simulink model "main_sim_adapt"  (Simulink 7.2)
settings: Solver=ode2  SolverMode=SingleTasking  StartTime=0.0  StopTime=tsim_max  FixedStep=dtsim  RelTol=1e-3
StopFcn:
  | %mkplt
undefined symbols (not defined in the file): aero_surf_qbar_off, aero_surf_qbar_on, assertion_time, att_type, att_type_numbers, bb_ellipsoid, bb_params, compute_all_rate_cols, compute_all_vel_cols, constants, cosA, DiscIntNeverNeededParam, dtsim, E_rwy, eow_boundary, full_surf_llim, full_surf_ulim, gain_set, gain_var_struct, in_exsig_vecin, in_exsig_vecout, MACH, MACH_att_fb, MACH_gain_mat, MACH_mass_IC, MACH_pos_IC, MACH_pqr_Bmat_IC, MACH_pqr_IC, MACH_pqr_u_IC, MACH_quat_IC, MACH_throttle_IC, MACH_U_nom_IC, MACH_vel_Bmat_IC, MACH_vel_cvdnom_IC, MACH_vel_IC, MACH_vel_uold_IC, max_LOS_rate, modes, N_rwy, pos, rcs_cvddes_thresh, reset_camcmd_on_entry, sinA, target_pos_IC, target_range_blind, target_range_detect, target_range_homing, target_vel_IC, trac_params, u_llim, u_ulim, use_auto_att_type, use_eow_as_iv, use_nav, use_pos_fltpath_lim, use_throt_estimate, use_variable_mass, use_wind_est, vel, vel_cmd_ramp_time ... (+1)
libraries: simulink x32, mach_lib x26, utility_lib x24, model_lib x15, simulink_need_slupdate x8, models x6
(part 1 of 5)
CloseFcn:
  | rtwprivate ssgencode ModelCloseRequest main
settings Model: Creator=E183308  LastModifiedBy=E183308  ModifiedComment=E700252 -- Tue Nov 11 13:33:23 2003 -- Version 1.2477  TunableVars=MACH_U_nom_IC,MACH_gain_mat,MACH_mass_IC,MACH_pos_IC,MACH_pqr_Bmat_IC,MACH_pqr_u_IC,MACH_quat_IC,MACH_throttle_IC,MACH_vel_Bmat_IC,MACH_vel_IC,MACH_vel_cvdnom_IC,MACH_vel_uold_IC  TunableVarsStorageClass=Auto,Auto,Auto,Auto,Auto,Auto,Auto,Auto,Auto,Auto,Auto,Auto  TunableVarsTypeQualifier=,,,,,,,,,,,  BufferReuse=off
settings DataIOCC: LimitDataPoints=off  SaveOutput=off  SaveTime=off  SignalLoggingName=sigsOut
settings OptimizationCC: BlockReduction=off  BooleanDataType=off  BufferReuse=off  EnforceIntegerDowncast=off  FoldNonRolledExpr=off  InitFltsAndDblsToZero=on
settings DebuggingCC: SaveWithParameterizedLinksMsg=none  SignalResolutionControl=TryResolveAllWithWarning  SolverPrmCheckMsg=none  InheritedTsInSrcMsg=none  MultiTaskDSMMsg=warning  MultiTaskCondExecSysMsg=none  StrictBusMsg=ErrorLevel1
settings HardwareCC: TargetEndianess=LittleEndian  TargetHWDeviceType=MATLAB Host  ProdEqTarget=off
settings SFSimCC: SFSimEcho=off
settings RTWCC: SystemTargetFile=rtwsfcn.tlc  TemplateMakefile=rtwsfcn_default_tmf  Description=S-function Target  ProcessScript=rtwsfcn_make_rtw_hook  IncludeERTFirstTime=on
settings STFCustomTargetCC: TargetFcnLib=ansi_tfl_tmw.mat  ModelReferenceCompliant=off  SystemTargetFile=rtwsfcn.tlc
settings CustomProperty: Value=on

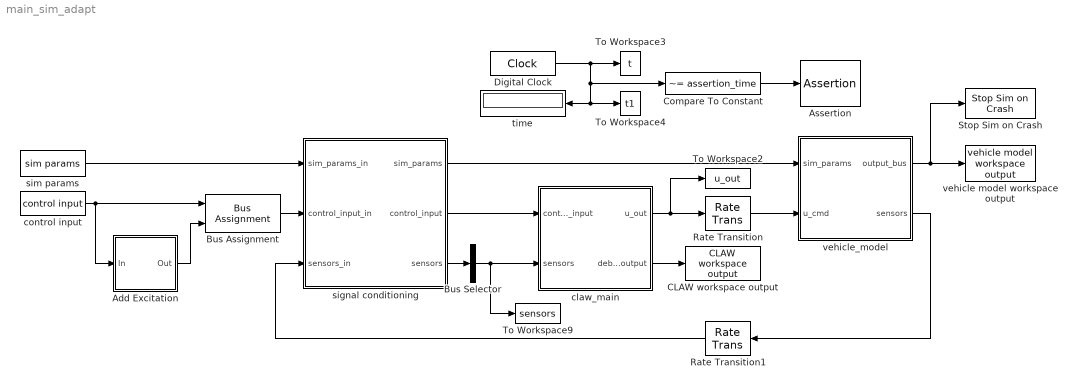
== system main_sim_adapt ==
  Add Excitation : Subsystem
  Assertion : Assertion  Enabled=on  AssertionFailFcn=assertioncb  StopWhenAssertionFail=off
  Bus Assignment : BusAssignment  AssignedSignals=command
  Bus Selector : BusSelector  OutputSignals=pqr,NED_dot,latlonh,e,accels_cg,nav_ok,u_meas,NED_wind,seeker  OutputAsBus=on
  CLAW workspace output : mach_lib/CLAW workspace output  SystemSampleTime=-1
  Compare To Constant : simulink/Logic and Bit Operations/Compare To Constant  SystemSampleTime=-1  relop=~=  const=assertion_time  LogicOutDataTypeMode=boolean  ZeroCross=off
  Digital Clock : DigitalClock  SampleTime=dtsim
  Rate Transition : RateTransition  X0=MACH_U_nom_IC
  Rate Transition1 : RateTransition  Orientation=left  OutPortSampleTime=MACH.dt
  Stop Sim on Crash : mach_lib/Stop Sim on Crash  SystemSampleTime=-1
  To Workspace2 : ToWorkspace  VariableName=u_out  SampleTime=MACH.dt  SaveFormat=Array
  To Workspace3 : ToWorkspace  VariableName=t  SampleTime=dtsim  SaveFormat=Array
  To Workspace4 : ToWorkspace  VariableName=t1  SampleTime=MACH.dt  SaveFormat=Array
  To Workspace9 : ToWorkspace  VariableName=sensors  SampleTime=MACH.dt  SaveFormat=Array
      settings: MaxDataPoints=1
  claw_main : Subsystem  AncestorBlock=mach_lib/claw_main  TreatAsAtomicUnit=on  SystemSampleTime=MACH.dt
  control input : mach_lib/control input  SystemSampleTime=MACH.dt
  signal conditioning : Subsystem
  sim params : mach_lib/sim params  SystemSampleTime=-1
  time : Display
  vehicle model workspace output : mach_lib/vehicle model workspace output  SystemSampleTime=-1
  vehicle_model : Subsystem  TreatAsAtomicUnit=on
  wires:
  Digital Clock/1 -> To Workspace3/1, time/1, To Workspace4/1, Compare To Constant/1
  claw_main/1(u_out) -> Rate Transition/1, To Workspace2/1
  vehicle_model/2(sensors) -> Rate Transition1/1
  claw_main/2(debug_output) -> CLAW workspace output/1
  Rate Transition/1 -> vehicle_model/2(u_cmd)
  Bus Selector/1 -> To Workspace9/1, claw_main/2(sensors)
  vehicle_model/1(output_bus) -> vehicle model workspace output/1, Stop Sim on Crash/1
  Rate Transition1/1 -> signal conditioning/3(sensors_in)
  signal conditioning/3(sensors) -> Bus Selector/1
  signal conditioning/2(control_input) -> claw_main/1(control_input)
  control input/1 -> Bus Assignment/1, Add Excitation/1(In)
  sim params/1 -> signal conditioning/1(sim_params_in)
  signal conditioning/1(sim_params) -> vehicle_model/1(sim_params)
  Compare To Constant/1 -> Assertion/1
  Bus Assignment/1 -> signal conditioning/2(control_input_in)
  Add Excitation/1(Out) -> Bus Assignment/2

== system main_sim_adapt/Add Excitation ==
  In : Inport
  Bus Selector1 : BusSelector  OutputSignals=command
      settings: CopyFcn=set_param(gcbh,'ShowName','off','CopyFcn','')
  Demux : Demux  Outputs=[1 1 1 1]
      settings: CopyFcn=set_param(gcbh,'ShowName','off','CopyFcn','')
  Excitation  Signal : Subsystem
  Mux : Mux
      settings: CopyFcn=set_param(gcbh,'ShowName','off','CopyFcn','')
  Rate Transition2 : RateTransition  OutPortSampleTime=MACH.dt
  Step : Step  SampleTime=MACH.dt
  Sum : Sum  Inputs=|++  OutDataType=sfix(16)  OutScaling=2^0
      settings: CopyFcn=set_param(gcbh,'ShowName','off','CopyFcn','')
  Out : Outport
  wires:
  Bus Selector1/1 -> Demux/1  "<command>"
  Demux/1 -> Mux/1
  Demux/3 -> Mux/3
  Demux/2 -> Sum/1
  Sum/1 -> Mux/2
  Step/1 -> Excitation  Signal/Enable
  Excitation  Signal/1(exsig) -> Rate Transition2/1
  Rate Transition2/1 -> Sum/2
  Demux/4 -> Mux/4
  In/1 -> Bus Selector1/1
  Mux/1 -> Out/1

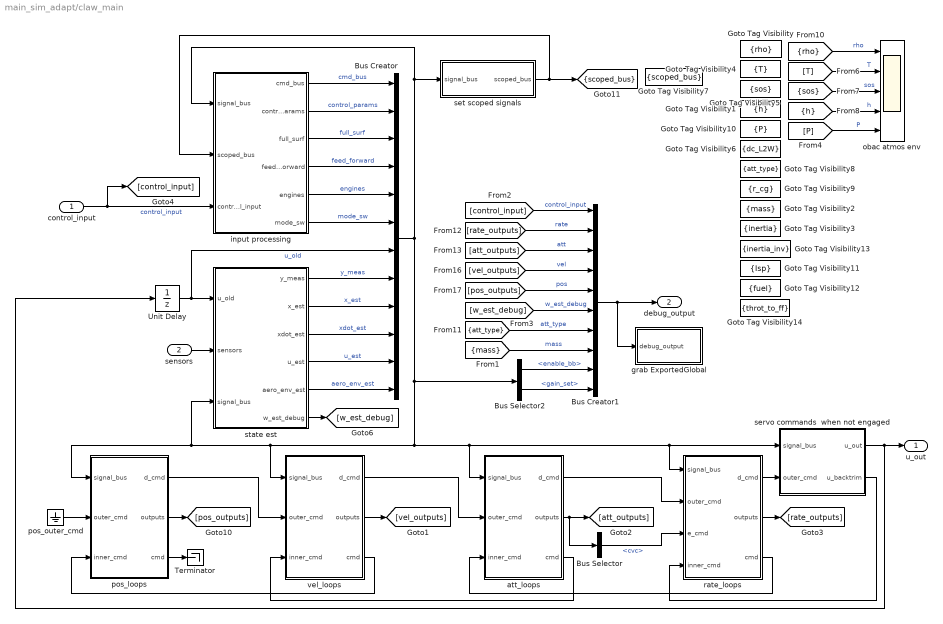
== system main_sim_adapt/claw_main ==
  control_input : Inport  OutDataType=sfix(16)  OutScaling=2^0
      settings: BusObject=control_input_bus
  sensors : Inport  Port=2  OutDataType=sfix(16)  OutScaling=2^0
  Bus Creator : BusCreator  Inputs=12
  Bus Creator1 : BusCreator  Inputs=10
      settings: BusObject=CLAW_DEBUG_OUTPUT_BUS
  Bus Selector : BusSelector  OutputSignals=cvc
  Bus Selector2 : BusSelector  OutputSignals=control_params.enable_bb,control_params.gain_set
  Goto Tag Visibility : GotoTagVisibility  GotoTag=rho
  Goto Tag Visibility1 : GotoTagVisibility  GotoTag=h
  Goto Tag Visibility10 : GotoTagVisibility  GotoTag=P
  Goto Tag Visibility11 : GotoTagVisibility  GotoTag=Isp
  Goto Tag Visibility12 : GotoTagVisibility  GotoTag=fuel
  Goto Tag Visibility13 : GotoTagVisibility  GotoTag=inertia_inv
  Goto Tag Visibility14 : GotoTagVisibility  GotoTag=throt_to_ff
  Goto Tag Visibility2 : GotoTagVisibility  GotoTag=mass
  Goto Tag Visibility3 : GotoTagVisibility  GotoTag=inertia
  Goto Tag Visibility4 : GotoTagVisibility  GotoTag=T
  Goto Tag Visibility5 : GotoTagVisibility  GotoTag=sos
  Goto Tag Visibility6 : GotoTagVisibility  GotoTag=dc_L2W
  Goto Tag Visibility7 : GotoTagVisibility  GotoTag=scoped_bus
  Goto Tag Visibility8 : GotoTagVisibility  GotoTag=att_type
  Goto Tag Visibility9 : GotoTagVisibility  GotoTag=r_cg
  Terminator : Terminator
  Unit Delay : UnitDelay  X0=MACH_U_nom_IC  SampleTime=-1
  att_loops : Subsystem
  grab ExportedGlobal : Subsystem
  input processing : Subsystem
  obac atmos env : Scope  NumInputPorts=5
      settings: YMin=-5~-5~-5~-5~-5  YMax=5~5~5~5~5  SaveName=ScopeData2
  pos_loops : Subsystem
      settings: RTWSystemCode=Function
  pos_outer_cmd : Ground
  rate_loops : Subsystem
      settings: RTWSystemCode=Function
  servo commands  when not engaged : Subsystem
  set scoped signals : Subsystem
  state est : Subsystem
  vel_loops : Subsystem
      settings: RTWSystemCode=Function
  u_out : Outport  OutDataType=sfix(16)  OutScaling=2^0
  debug_output : Outport  Port=2  OutDataType=sfix(16)  OutScaling=2^0
  tag scope: scoped_bus=scoped
  wires:
  input processing/6(mode_sw) -> Bus Creator/6  "mode_sw"
  input processing/5(engines) -> Bus Creator/5  "engines"
  pos_loops/2(outputs) -> [pos_outputs]
  [pos_outputs] -> Bus Creator1/5  "pos"
  [vel_outputs] -> Bus Creator1/4  "vel"
  [att_outputs] -> Bus Creator1/3  "att"
  [rate_outputs] -> Bus Creator1/2  "rate"
  att_loops/1(d_cmd) -> rate_loops/2(outer_cmd)
  vel_loops/1(d_cmd) -> att_loops/2(outer_cmd)
  rate_loops/1(d_cmd) -> servo commands  when not engaged/2(outer_cmd)
  Bus Creator/1 -> att_loops/1(signal_bus), rate_loops/1(signal_bus), servo commands  when not engaged/1(signal_bus), vel_loops/1(signal_bus), pos_loops/1(signal_bus), state est/3(signal_bus), Bus Selector2/1, input processing/1(signal_bus), set scoped signals/1(signal_bus)
  pos_loops/3(cmd) -> Terminator/1
  att_loops/3(cmd) -> vel_loops/3(inner_cmd)
  rate_loops/3(cmd) -> att_loops/3(inner_cmd)
  pos_loops/1(d_cmd) -> vel_loops/2(outer_cmd)
  vel_loops/2(outputs) -> [vel_outputs]
  att_loops/2(outputs) -> [att_outputs], Bus Selector/1
  rate_loops/2(outputs) -> [rate_outputs]
  Bus Creator1/1 -> debug_output/1, grab ExportedGlobal/1(debug_output)
  Unit Delay/1 -> state est/1(u_old), Bus Creator/7  "u_old"
  sensors/1 -> state est/2(sensors)
  vel_loops/3(cmd) -> pos_loops/3(inner_cmd)
  servo commands  when not engaged/2(u_backtrim) -> rate_loops/4(inner_cmd)
  state est/4(u_est) -> Bus Creator/11  "u_est"
  state est/3(xdot_est) -> Bus Creator/10  "xdot_est"
  state est/2(x_est) -> Bus Creator/9  "x_est"
  state est/1(y_meas) -> Bus Creator/8  "y_meas"
  servo commands  when not engaged/1(u_out) -> u_out/1, Unit Delay/1
  pos_outer_cmd/1 -> pos_loops/2(outer_cmd)
  state est/6(w_est_debug) -> [w_est_debug]
  [w_est_debug] -> Bus Creator1/6  "w_est_debug"
  [att_type] -> Bus Creator1/7  "att_type"
  input processing/2(control_params) -> Bus Creator/2  "control_params"
  [h] -> obac atmos env/4  "h"
  [sos] -> obac atmos env/3  "sos"
  [T] -> obac atmos env/2  "T"
  [rho] -> obac atmos env/1  "rho"
  [P] -> obac atmos env/5  "P"
  state est/5(aero_env_est) -> Bus Creator/12  "aero_env_est"
  input processing/3(full_surf) -> Bus Creator/3  "full_surf"
  input processing/4(feed_forward) -> Bus Creator/4  "feed_forward"
  set scoped signals/1(scoped_bus) -> [scoped_bus], input processing/2(scoped_bus)
  [mass] -> Bus Creator1/8  "mass"
  Bus Selector2/1 -> Bus Creator1/9  "<enable_bb>"
  Bus Selector2/2 -> Bus Creator1/10  "<gain_set>"
  control_input/1 -> input processing/3(control_input), [control_input]  "control_input"
  input processing/1(cmd_bus) -> Bus Creator/1  "cmd_bus"
  [control_input] -> Bus Creator1/1  "control_input"
  Bus Selector/1 -> rate_loops/3(e_cmd)  "<cvc>"

== system main_sim_adapt/signal conditioning ==
  sim_params_in : Inport  OutDataType=sfix(16)  OutScaling=2^0
  control_input_in : Inport  Port=2  OutDataType=sfix(16)  OutScaling=2^0
  sensors_in : Inport  Port=3  OutDataType=sfix(16)  OutScaling=2^0
  Bus Assignment : BusAssignment  AssignedSignals=full_surf.full_surf_pref
  Bus Selector : BusSelector  OutputSignals=full_surf.full_surf_pref
  Compare To Constant : simulink/Logic and Bit Operations/Compare To Constant  SystemSampleTime=-1  relop=>=  const=0  LogicOutDataTypeMode=boolean  ZeroCross=off
  Compare To Constant1 : simulink/Logic and Bit Operations/Compare To Constant  SystemSampleTime=-1  relop=<=  const=5  LogicOutDataTypeMode=boolean  ZeroCross=off
  Constant : Constant  Value=360  OutDataType=sfix(16)  OutScaling=2^0
  Digital Clock : DigitalClock  SampleTime=MACH.dt
  Gain : Gain  Gain=0  ParameterDataType=sfix(16)  ParameterScaling=2^0  OutDataType=sfix(16)  OutScaling=2^0
  Logical Operator : Logic  AllPortsSameDT=off
  Product : Product  OutDataType=sfix(16)  OutScaling=2^0  RndMeth=Zero
  Sine Wave : Sin  TimeSource=Use external signal  Amplitude=5  Frequency=2*pi  SampleTime=0
  Sum : Sum  Inputs=|++  OutDataType=sfix(16)  OutScaling=2^0
  Sum1 : Sum  Inputs=|+-  OutDataType=sfix(16)  OutScaling=2^0
  get RIE : Selector  InputPortWidth=MACH.num_u  IndexOptions=Index vector (dialog)  Indices=MACH.vane_idx(1)  OutputSizes=1
  set RIE : Assignment  IndexOptions=Index vector (dialog)  Indices=MACH.vane_idx(1)  OutputSizes=[1 1]
  sim_params : Outport  OutDataType=sfix(16)  OutScaling=2^0
  control_input : Outport  Port=2  OutDataType=sfix(16)  OutScaling=2^0
  sensors : Outport  Port=3  OutDataType=sfix(16)  OutScaling=2^0
  wires:
  sim_params_in/1 -> sim_params/1
  control_input_in/1 -> Bus Assignment/1, Bus Selector/1
  sensors_in/1 -> sensors/1
  set RIE/1 -> Bus Assignment/2
  Sum/1 -> set RIE/2
  Bus Selector/1 -> set RIE/1, get RIE/1  "<full_surf_pref>"
  get RIE/1 -> Sum/1
  Digital Clock/1 -> Sum1/1
  Constant/1 -> Sum1/2
  Sum1/1 -> Sine Wave/1, Compare To Constant/1, Compare To Constant1/1
  Compare To Constant/1 -> Logical Operator/1
  Compare To Constant1/1 -> Logical Operator/2
  Logical Operator/1 -> Product/2
  Sine Wave/1 -> Product/1
  Product/1 -> Gain/1
  Bus Assignment/1 -> control_input/1
  Gain/1 -> Sum/2

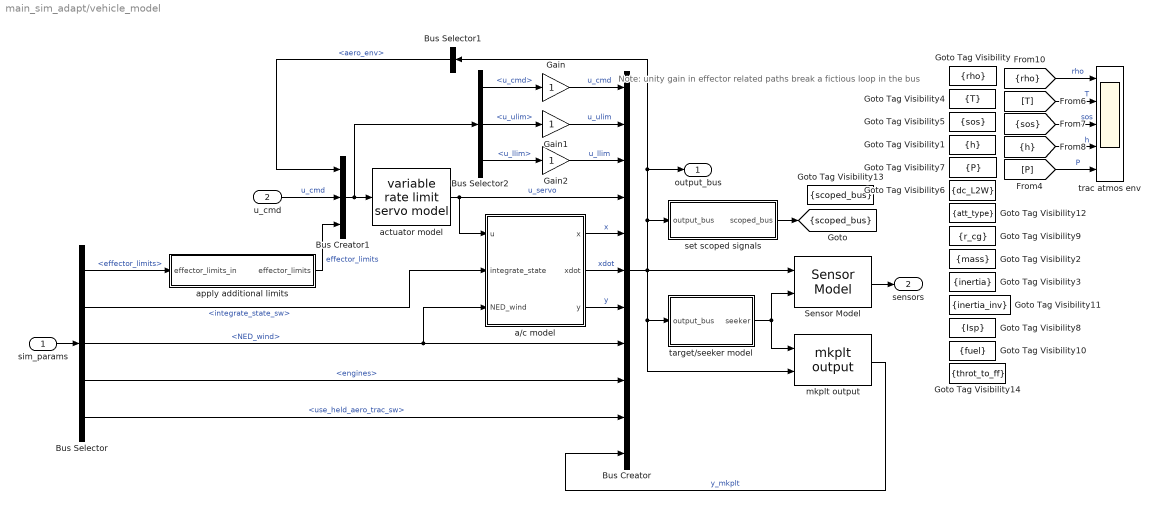
== system main_sim_adapt/vehicle_model ==
  note: Note: unity gain in effector related paths
      | break a fictious loop in the bus
  sim_params : Inport  OutDataType=sfix(16)  OutScaling=2^0
  u_cmd : Inport  Port=2  OutDataType=sfix(16)  OutScaling=2^0
  Bus Creator : BusCreator  Inputs=11
  Bus Creator1 : BusCreator  Inputs=3
  Bus Selector : BusSelector  OutputSignals=effector_limits,integrate_state_sw,NED_wind,engines,use_held_aero_trac_sw
  Bus Selector1 : BusSelector  Orientation=left  OutputSignals=y.aero_env
  Bus Selector2 : BusSelector  OutputSignals=u_cmd,effector_limits.u_ulim,effector_limits.u_llim
  Gain : Gain  ParameterDataType=sfix(16)  ParameterScaling=2^0  OutDataType=sfix(16)  OutScaling=2^0
  Gain1 : Gain  ParameterDataType=sfix(16)  ParameterScaling=2^0  OutDataType=sfix(16)  OutScaling=2^0
  Gain2 : Gain  ParameterDataType=sfix(16)  ParameterScaling=2^0  OutDataType=sfix(16)  OutScaling=2^0
  Goto Tag Visibility : GotoTagVisibility  GotoTag=rho
  Goto Tag Visibility1 : GotoTagVisibility  GotoTag=h
  Goto Tag Visibility10 : GotoTagVisibility  GotoTag=fuel
  Goto Tag Visibility11 : GotoTagVisibility  GotoTag=inertia_inv
  Goto Tag Visibility12 : GotoTagVisibility  GotoTag=att_type
  Goto Tag Visibility13 : GotoTagVisibility  GotoTag=scoped_bus
  Goto Tag Visibility14 : GotoTagVisibility  GotoTag=throt_to_ff
  Goto Tag Visibility2 : GotoTagVisibility  GotoTag=mass
  Goto Tag Visibility3 : GotoTagVisibility  GotoTag=inertia
  Goto Tag Visibility4 : GotoTagVisibility  GotoTag=T
  Goto Tag Visibility5 : GotoTagVisibility  GotoTag=sos
  Goto Tag Visibility6 : GotoTagVisibility  GotoTag=dc_L2W
  Goto Tag Visibility7 : GotoTagVisibility  GotoTag=P
  Goto Tag Visibility8 : GotoTagVisibility  GotoTag=Isp
  Goto Tag Visibility9 : GotoTagVisibility  GotoTag=r_cg
  Sensor Model : model_lib/Sensor Model  SystemSampleTime=-1
  a/c model : Subsystem
  actuator model : model_lib/variable rate limit servo model  SystemSampleTime=-1
  apply additional limits : Subsystem
  mkplt output : model_lib/mkplt output  SystemSampleTime=-1
  set scoped signals : Subsystem
  target/seeker model : Subsystem
  trac atmos env : Scope  NumInputPorts=5
      settings: YMin=-5~-5~-5~-5~-5  YMax=5~5~5~5~5
  output_bus : Outport  OutDataType=sfix(16)  OutScaling=2^0
  sensors : Outport  Port=2  OutDataType=sfix(16)  OutScaling=2^0
  tag scope: scoped_bus=scoped
  wires:
  actuator model/1 -> a/c model/1(u), Bus Creator/4  "u_servo"
  Sensor Model/1 -> sensors/1
  Bus Selector/3 -> Bus Creator/8, a/c model/3(NED_wind)  "<NED_wind>"
  [h] -> trac atmos env/4  "h"
  [sos] -> trac atmos env/3  "sos"
  [T] -> trac atmos env/2  "T"
  [rho] -> trac atmos env/1  "rho"
  [P] -> trac atmos env/5  "P"
  target/seeker model/1(seeker) -> Sensor Model/2, mkplt output/1
  a/c model/1(x) -> Bus Creator/5  "x"
  a/c model/2(xdot) -> Bus Creator/6  "xdot"
  a/c model/3(y) -> Bus Creator/7  "y"
  Bus Creator/1 -> set scoped signals/1(output_bus), output_bus/1, Bus Selector1/1, target/seeker model/1(output_bus), mkplt output/2, Sensor Model/1
  sim_params/1 -> Bus Selector/1
  set scoped signals/1(scoped_bus) -> [scoped_bus]
  Bus Selector/4 -> Bus Creator/9  "<engines>"
  mkplt output/1 -> Bus Creator/11  "y_mkplt"
  Bus Selector/5 -> Bus Creator/10  "<use_held_aero_trac_sw>"
  Bus Creator1/1 -> actuator model/1, Bus Selector2/1
  Bus Selector1/1 -> Bus Creator1/1  "<aero_env>"
  u_cmd/1 -> Bus Creator1/2  "u_cmd"
  Bus Selector2/1 -> Gain/1  "<u_cmd>"
  Bus Selector2/2 -> Gain1/1  "<u_ulim>"
  Bus Selector2/3 -> Gain2/1  "<u_llim>"
  Gain/1 -> Bus Creator/1  "u_cmd"
  Gain1/1 -> Bus Creator/2  "u_ulim"
  Gain2/1 -> Bus Creator/3  "u_llim"
  Bus Selector/2 -> a/c model/2(integrate_state)  "<integrate_state_sw>"
  Bus Selector/1 -> apply additional limits/1(effector_limits_in)  "<effector_limits>"
  apply additional limits/1(effector_limits) -> Bus Creator1/3  "effector_limits"

== system main_sim_adapt/Add Excitation/Excitation  Signal ==
  Enable : EnablePort  StatesWhenEnabling=reset  ShowOutputPort=on
  Integrator : Integrator  ExternalReset=falling
  Lookup Table1 : Lookup  InputValues=in_exsig_vecin  Table=in_exsig_vecout  LookUpMeth=Use Input Above  OutDataType=sfix(16)  OutScaling=2^0
  excitaiton output sig : Scope
      settings: TimeRange=45  YMin=-0.05  YMax=0.05  SaveName=ScopeData5
  excitation input sig : Scope
      settings: TimeRange=45  YMin=15  YMax=22  SaveName=ScopeData10
  exsig : Outport  OutDataType=sfix(16)  OutScaling=2^0  OutputWhenDisabled=reset  InitialOutput=0
  wires:
  Lookup Table1/1 -> exsig/1, excitaiton output sig/1
  Enable/1 -> Integrator/1, Integrator/2
  Integrator/1 -> Lookup Table1/1, excitation input sig/1

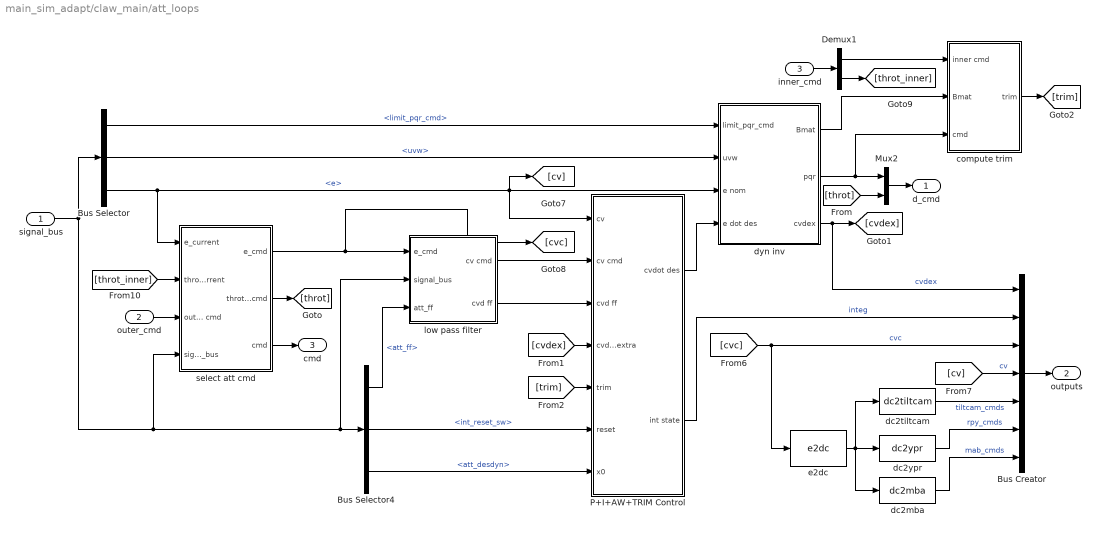
== system main_sim_adapt/claw_main/att_loops ==
  signal_bus : Inport  OutDataType=sfix(16)  OutScaling=2^0
  outer_cmd : Inport  Port=2  OutDataType=sfix(16)  OutScaling=2^0
  inner_cmd : Inport  Port=3  OutDataType=sfix(16)  OutScaling=2^0
  Bus Creator : BusCreator  Inputs=7
  Bus Selector : BusSelector  OutputSignals=control_params.limit_pqr_cmd,x_est.uvw,x_est.e
  Bus Selector4 : BusSelector  OutputSignals=feed_forward.att_ff,mode_sw.int_reset_sw,control_params.att_desdyn
  Demux1 : Demux  Outputs=[ MACH.att_num_u MACH.num_u_throt ]
  Mux2 : Mux  Inputs=2
  P+I+AW+TRIM Control : Subsystem
  compute trim : Subsystem
  dc2mba : utility_lib/dc2mba  SystemSampleTime=-1
  dc2tiltcam : utility_lib/dc2tiltcam  SystemSampleTime=-1
  dc2ypr : utility_lib/dc2ypr  SystemSampleTime=-1
  dyn inv : Subsystem
  e2dc : utility_lib/e2dc  SystemSampleTime=-1
  low pass filter : Subsystem
  select att cmd : Subsystem
  d_cmd : Outport  OutDataType=sfix(16)  OutScaling=2^0
  outputs : Outport  Port=2  OutDataType=sfix(16)  OutScaling=2^0
  cmd : Outport  Port=3  OutDataType=sfix(16)  OutScaling=2^0
  wires:
  Mux2/1 -> d_cmd/1
  [throt] -> Mux2/2
  P+I+AW+TRIM Control/2(int state) -> Bus Creator/2  "integ"
  dyn inv/3(cvdex) -> [cvdex], Bus Creator/1  "cvdex"
  Bus Selector/3 -> select att cmd/1(e_current), dyn inv/3(e nom), [cv], P+I+AW+TRIM Control/1(cv)  "<e>"
  outer_cmd/1 -> select att cmd/3(outer cmd)
  P+I+AW+TRIM Control/1(cvdot des) -> dyn inv/4(e dot des)
  [cvdex] -> P+I+AW+TRIM Control/4(cvdot extra)
  dyn inv/1(Bmat) -> compute trim/2(Bmat)
  [trim] -> P+I+AW+TRIM Control/5(trim)
  signal_bus/1 -> Bus Selector/1, select att cmd/4(signal_bus), Bus Selector4/1, low pass filter/2(signal_bus)
  compute trim/1(trim) -> [trim]
  select att cmd/2(throt_cmd) -> [throt]
  [cvc] -> Bus Creator/3, e2dc/1  "cvc"
  Bus Creator/1 -> outputs/1
  inner_cmd/1 -> Demux1/1
  Demux1/1 -> compute trim/1(inner cmd)
  Demux1/2 -> [throt_inner]
  dc2tiltcam/1 -> Bus Creator/5  "tiltcam_cmds"
  [cv] -> Bus Creator/4  "cv"
  e2dc/1 -> dc2tiltcam/1, dc2ypr/1, dc2mba/1
  dc2ypr/1 -> Bus Creator/6  "rpy_cmds"
  dc2mba/1 -> Bus Creator/7  "mab_cmds"
  Bus Selector/2 -> dyn inv/2(uvw)  "<uvw>"
  Bus Selector4/3 -> P+I+AW+TRIM Control/7(x0)  "<att_desdyn>"
  select att cmd/3(cmd) -> cmd/1
  dyn inv/2(pqr) -> Mux2/1, compute trim/3(cmd)
  Bus Selector4/2 -> P+I+AW+TRIM Control/6(reset)  "<int_reset_sw>"
  Bus Selector/1 -> dyn inv/1(limit_pqr_cmd)  "<limit_pqr_cmd>"
  [throt_inner] -> select att cmd/2(throt_current)
  select att cmd/1(e_cmd) -> low pass filter/1(e_cmd), [cvc]
  low pass filter/1(cv cmd) -> P+I+AW+TRIM Control/2(cv cmd)
  low pass filter/2(cvd ff) -> P+I+AW+TRIM Control/3(cvd ff)
  Bus Selector4/1 -> low pass filter/3(att_ff)  "<att_ff>"

== system main_sim_adapt/claw_main/grab ExportedGlobal ==
  debug_output : Inport  OutDataType=sfix(16)  OutScaling=2^0
  Terminator{1..4,6} (5 alike) : Terminator
  grab cv variables : Subsystem
  grab cvcmd variables : Subsystem
  grab cvdex variables : Subsystem
  grab integrator variables : Subsystem
  grab w_est variables : Subsystem
  wires:
  debug_output/1 -> grab cv variables/1(In1), grab w_est variables/1(In1), grab cvcmd variables/1(In1), grab integrator variables/1(In1), grab cvdex variables/1(In1)
  grab cvdex variables/1(Out1) -> Terminator1/1
  grab integrator variables/1(Out1) -> Terminator2/1
  grab cvcmd variables/1(Out1) -> Terminator3/1
  grab cv variables/1(Out1) -> Terminator4/1
  grab w_est variables/1(Out1) -> Terminator6/1

== system main_sim_adapt/claw_main/input processing ==
  signal_bus : Inport  OutDataType=sfix(16)  OutScaling=2^0
  scoped_bus : Inport  Port=2  OutDataType=sfix(16)  OutScaling=2^0
  control_input : Inport  Port=3  OutDataType=sfix(16)  OutScaling=2^0
  Bus Selector2 : BusSelector  OutputSignals=full_surf
  Bus Selector3 : BusSelector  OutputSignals=engines,mode_sw,command
  Bus Selector4 : BusSelector  OutputSignals=u_old,y_meas.u_meas
  mode dependent stick processing : Subsystem
  modify limits and apply to direct commands : Subsystem
  select att_type : Subsystem
  set control parameters : Subsystem
  cmd_bus : Outport  OutDataType=sfix(16)  OutScaling=2^0
  control_params : Outport  Port=2  OutDataType=sfix(16)  OutScaling=2^0
  full_surf : Outport  Port=3  OutDataType=sfix(16)  OutScaling=2^0
  feed_forward : Outport  Port=4  OutDataType=sfix(16)  OutScaling=2^0
  engines : Outport  Port=5  OutDataType=sfix(16)  OutScaling=2^0
  mode_sw : Outport  Port=6  OutDataType=sfix(16)  OutScaling=2^0
  wires:
  Bus Selector3/1 -> engines/1  "<engines>"
  mode dependent stick processing/1(cmd_bus) -> cmd_bus/1
  Bus Selector3/3 -> mode dependent stick processing/1(command)  "<command>"
  set control parameters/1(control_params) -> control_params/1
  Bus Selector4/1 -> modify limits and apply to direct commands/1(u_old)  "<u_old>"
  Bus Selector2/1 -> modify limits and apply to direct commands/3(full_surf_in)  "<full_surf>"
  modify limits and apply to direct commands/1(full_surf) -> full_surf/1, set control parameters/2(full_surf)
  control_input/1 -> Bus Selector3/1, Bus Selector2/1
  signal_bus/1 -> set control parameters/1(signal_bus), Bus Selector4/1, mode dependent stick processing/2(signal_bus), select att_type/3(signal_bus)
  mode dependent stick processing/2(feed_forward) -> feed_forward/1
  Bus Selector3/2 -> select att_type/2(mode_sw_in)  "<mode_sw>"
  scoped_bus/1 -> select att_type/1(scoped_bus)
  select att_type/1(mode_sw) -> mode_sw/1
  Bus Selector4/2 -> modify limits and apply to direct commands/2(u_meas)  "<u_meas>"

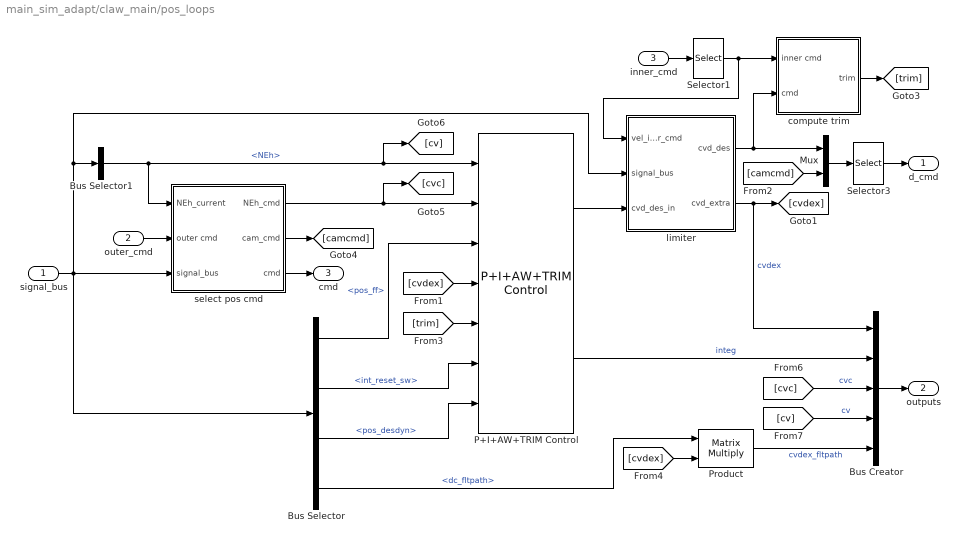
== system main_sim_adapt/claw_main/pos_loops ==
  signal_bus : Inport  OutDataType=sfix(16)  OutScaling=2^0
  outer_cmd : Inport  Port=2  OutDataType=sfix(16)  OutScaling=2^0
  inner_cmd : Inport  Port=3  OutDataType=sfix(16)  OutScaling=2^0
  Bus Creator : BusCreator  Inputs=5
  Bus Selector : BusSelector  OutputSignals=feed_forward.pos_ff,mode_sw.int_reset_sw,control_params.pos_desdyn,y_meas.dc_fltpath
  Bus Selector1 : BusSelector  OutputSignals=x_est.NEh
  Mux : Mux  Inputs=[3 1 ]
  P+I+AW+TRIM Control : mach_lib/P+I+AW+TRIM Control  SystemSampleTime=-1
  Product : Product  Multiplication=Matrix(*)  OutDataType=sfix(16)  OutScaling=2^0  RndMeth=Zero
  Selector1 : Selector  InputPortWidth=4  IndexOptions=Index vector (dialog)  Indices=[1 2 4]  OutputSizes=1
  Selector3 : Selector  InputPortWidth=4  IndexOptions=Index vector (dialog)  Indices=[1 2 4 3]  OutputSizes=1
  compute trim : Subsystem
  limiter : Subsystem
  select pos cmd : Subsystem
  d_cmd : Outport  OutDataType=sfix(16)  OutScaling=2^0
  outputs : Outport  Port=2  OutDataType=sfix(16)  OutScaling=2^0
  cmd : Outport  Port=3  OutDataType=sfix(16)  OutScaling=2^0
  wires:
  [camcmd] -> Mux/2
  Mux/1 -> Selector3/1
  select pos cmd/1(NEh_cmd) -> P+I+AW+TRIM Control/2, [cvc]
  Bus Selector1/1 -> P+I+AW+TRIM Control/1, [cv], select pos cmd/1(NEh_current)  "<NEh>"
  signal_bus/1 -> Bus Selector/1, select pos cmd/3(signal_bus), Bus Selector1/1, limiter/2(signal_bus)
  compute trim/1(trim) -> [trim]
  inner_cmd/1 -> Selector1/1
  Selector1/1 -> compute trim/1(inner cmd), limiter/1(vel_inner_cmd)
  outer_cmd/1 -> select pos cmd/2(outer cmd)
  select pos cmd/3(cmd) -> cmd/1
  Selector3/1 -> d_cmd/1
  [cvc] -> Bus Creator/3  "cvc"
  [cv] -> Bus Creator/4  "cv"
  [trim] -> P+I+AW+TRIM Control/5
  [cvdex] -> P+I+AW+TRIM Control/4
  Bus Selector/2 -> P+I+AW+TRIM Control/6  "<int_reset_sw>"
  Bus Selector/3 -> P+I+AW+TRIM Control/7  "<pos_desdyn>"
  limiter/1(cvd_des) -> Mux/1, compute trim/2(cmd)
  P+I+AW+TRIM Control/1 -> limiter/3(cvd_des_in)
  [cvdex] -> Product/2
  P+I+AW+TRIM Control/2 -> Bus Creator/2  "integ"
  Bus Creator/1 -> outputs/1
  Bus Selector/4 -> Product/1  "<dc_fltpath>"
  Product/1 -> Bus Creator/5  "cvdex_fltpath"
  limiter/2(cvd_extra) -> Bus Creator/1, [cvdex]  "cvdex"
  Bus Selector/1 -> P+I+AW+TRIM Control/3  "<pos_ff>"
  select pos cmd/2(cam_cmd) -> [camcmd]

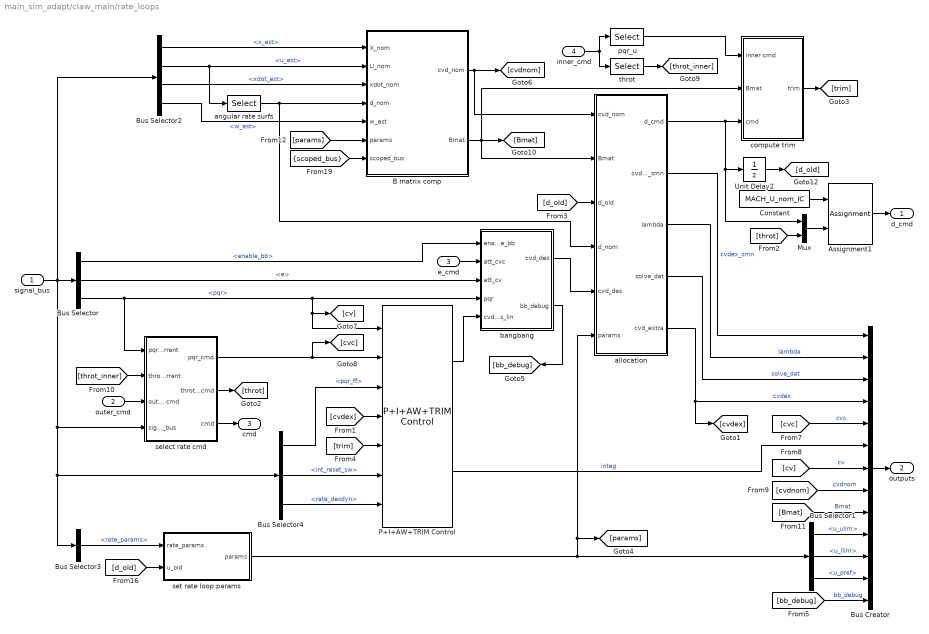
== system main_sim_adapt/claw_main/rate_loops ==
  signal_bus : Inport  OutDataType=sfix(16)  OutScaling=2^0
  outer_cmd : Inport  Port=2  OutDataType=sfix(16)  OutScaling=2^0
  e_cmd : Inport  Port=3  OutDataType=sfix(16)  OutScaling=2^0
  inner_cmd : Inport  Port=4  OutDataType=sfix(16)  OutScaling=2^0
  Assignment1 : Assignment  IndexOptions=Index vector (dialog)  Indices=[MACH.pqr_u_idx MACH.throttle_idx]  OutputSizes=[1 1]
  B matrix comp : Subsystem  TreatAsAtomicUnit=on
  Bus Creator : BusCreator  Inputs=13
  Bus Selector : BusSelector  OutputSignals=control_params.enable_bb,x_est.e,x_est.pqr
  Bus Selector1 : BusSelector  OutputSignals=u_ulim,u_llim,u_pref
  Bus Selector2 : BusSelector  OutputSignals=x_est,u_est,xdot_est,y_meas.w_est
  Bus Selector3 : BusSelector  OutputSignals=control_params.rate_params
  Bus Selector4 : BusSelector  OutputSignals=feed_forward.pqr_ff,mode_sw.int_reset_sw,control_params.rate_desdyn
  Constant : Constant  Value=MACH_U_nom_IC  OutDataType=sfix(16)  OutScaling=2^0
  Mux : Mux  Inputs=2
  P+I+AW+TRIM Control : mach_lib/P+I+AW+TRIM Control  SystemSampleTime=-1
  Unit Delay2 : UnitDelay  X0=MACH_pqr_u_IC  SampleTime=-1
  allocation : Subsystem
  angular rate surfs : Selector  InputPortWidth=MACH.num_u  IndexOptions=Index vector (dialog)  Indices=MACH.pqr_u_idx  OutputSizes=1
  bangbang : Subsystem
  compute trim : Subsystem
  pqr_u : Selector  InputPortWidth=MACH.num_u  IndexOptions=Index vector (dialog)  Indices=MACH.pqr_u_idx  OutputSizes=1
  select rate cmd : Subsystem
  set rate loop params : Subsystem
  throt : Selector  InputPortWidth=MACH.num_u  IndexOptions=Index vector (dialog)  Indices=MACH.throttle_idx  OutputSizes=1
  d_cmd : Outport  OutDataType=sfix(16)  OutScaling=2^0
  outputs : Outport  Port=2  OutDataType=sfix(16)  OutScaling=2^0
  cmd : Outport  Port=3  OutDataType=sfix(16)  OutScaling=2^0
  wires:
  angular rate surfs/1 -> B matrix comp/4(d_nom), allocation/4(d_nom)
  outer_cmd/1 -> select rate cmd/3(outer cmd)
  B matrix comp/1(cvd_nom) -> [cvdnom], allocation/1(cvd_nom)
  P+I+AW+TRIM Control/2 -> Bus Creator/6  "integ"
  signal_bus/1 -> Bus Selector2/1, Bus Selector/1, Bus Selector3/1, Bus Selector4/1, select rate cmd/4(signal_bus)
  compute trim/1(trim) -> [trim]
  inner_cmd/1 -> pqr_u/1, throt/1
  select rate cmd/2(throt_cmd) -> [throt]
  select rate cmd/1(pqr_cmd) -> [cvc], P+I+AW+TRIM Control/2
  [throt_inner] -> select rate cmd/2(throt_current)
  [cvc] -> Bus Creator/5  "cvc"
  [cv] -> Bus Creator/7  "cv"
  [cvdnom] -> Bus Creator/8  "cvdnom"
  set rate loop params/1(params) -> Bus Selector1/1, allocation/6(params), [params]
  Assignment1/1 -> d_cmd/1
  throt/1 -> [throt_inner]
  [trim] -> P+I+AW+TRIM Control/5
  [cvdex] -> P+I+AW+TRIM Control/4
  Bus Selector/3 -> select rate cmd/1(pqr_current), bangbang/4(pqr), P+I+AW+TRIM Control/1, [cv]  "<pqr>"
  Bus Selector4/1 -> P+I+AW+TRIM Control/3  "<pqr_ff>"
  Bus Selector4/2 -> P+I+AW+TRIM Control/6  "<int_reset_sw>"
  [Bmat] -> Bus Creator/9  "Bmat"
  Bus Selector1/1 -> Bus Creator/10  "<u_ulim>"
  Bus Selector1/2 -> Bus Creator/11  "<u_llim>"
  [d_old] -> set rate loop params/2(u_old)
  pqr_u/1 -> compute trim/1(inner cmd)
  Constant/1 -> Assignment1/1
  Mux/1 -> Assignment1/2
  Bus Selector2/1 -> B matrix comp/1(X_nom)  "<x_est>"
  Bus Selector2/2 -> angular rate surfs/1, B matrix comp/2(U_nom)  "<u_est>"
  Bus Selector2/3 -> B matrix comp/3(xdot_nom)  "<xdot_est>"
  Bus Selector2/4 -> B matrix comp/5(w_est)  "<w_est>"
  Bus Selector1/3 -> Bus Creator/12  "<u_pref>"
  allocation/5(cvd_extra) -> Bus Creator/4, [cvdex]  "cvdex"
  [throt] -> Mux/2
  Unit Delay2/1 -> [d_old]
  allocation/1(d_cmd) -> compute trim/3(cmd), Mux/1, Unit Delay2/1
  [d_old] -> allocation/3(d_old)
  B matrix comp/2(Bmat) -> compute trim/2(Bmat), [Bmat], allocation/2(Bmat)
  allocation/3(lambda) -> Bus Creator/2  "lambda"
  allocation/4(solve_dat) -> Bus Creator/3  "solve_dat"
  Bus Creator/1 -> outputs/1
  [scoped_bus] -> B matrix comp/7(scoped_bus)
  [params] -> B matrix comp/6(params)
  Bus Selector4/3 -> P+I+AW+TRIM Control/7  "<rate_desdyn>"
  allocation/2(cvd_extra_smn) -> Bus Creator/1  "cvdex_smn"
  bangbang/1(cvd_des) -> allocation/5(cvd_des)
  e_cmd/1 -> bangbang/2(att_cvc)
  Bus Selector/2 -> bangbang/3(att_cv)  "<e>"
  P+I+AW+TRIM Control/1 -> bangbang/5(cvd_des_lin)
  Bus Selector/1 -> bangbang/1(enable_bb)  "<enable_bb>"
  bangbang/2(bb_debug) -> [bb_debug]
  [bb_debug] -> Bus Creator/13  "bb_debug"
  select rate cmd/3(cmd) -> cmd/1
  Bus Selector3/1 -> set rate loop params/1(rate_params)  "<rate_params>"

== system main_sim_adapt/claw_main/servo commands  when not engaged ==
  note: for OAV/MAV during "pre-takeoff",
      |  the rate inner_cmd throt was set to takeoff throt
      | to allow integrators to trim for anticipated takeoff.
      | This should be revisited within current CLAW
      | before being used again.
  signal_bus : Inport  OutDataType=sfix(16)  OutScaling=2^0
  outer_cmd : Inport  Port=2  OutDataType=sfix(16)  OutScaling=2^0
  Bus Selector1 : BusSelector  OutputSignals=mode_sw.pre_takeoff_sw,mode_sw.engaged_sw,mode_sw.full_surf_cmd_sw,cmd_bus.autopilot_cmd,full_surf.full_surf_cmd
  Constant1 : Constant  Value=MACH.pre_takeoff_u_backtrim  OutDataType=sfix(16)  OutScaling=2^0
  Multiport Switch : MultiPortSwitch  Inputs=2  zeroidx=on
  Multiport Switch1 : MultiPortSwitch  Inputs=2  zeroidx=on
  Multiport Switch2 : MultiPortSwitch  Inputs=2  zeroidx=on
  pseudo surf cmd : Subsystem
  u_out : Outport  OutDataType=sfix(16)  OutScaling=2^0
  u_backtrim : Outport  Port=2  OutDataType=sfix(16)  OutScaling=2^0
  wires:
  signal_bus/1 -> Bus Selector1/1
  Bus Selector1/1 -> Multiport Switch/1  "<pre_takeoff_sw>"
  Multiport Switch1/1 -> Multiport Switch/2, u_out/1
  Constant1/1 -> Multiport Switch/3
  Bus Selector1/2 -> Multiport Switch1/1  "<engaged_sw>"
  Bus Selector1/3 -> Multiport Switch2/1  "<full_surf_cmd_sw>"
  Bus Selector1/4 -> pseudo surf cmd/1(autopilot_cmd)  "<autopilot_cmd>"
  pseudo surf cmd/1(surf_cmd) -> Multiport Switch2/2
  Bus Selector1/5 -> Multiport Switch2/3  "<full_surf_cmd>"
  Multiport Switch2/1 -> Multiport Switch1/2
  outer_cmd/1 -> Multiport Switch1/3
  Multiport Switch/1 -> u_backtrim/1

== system main_sim_adapt/claw_main/set scoped signals ==
  signal_bus : Inport  OutDataType=sfix(16)  OutScaling=2^0
  Bus Selector3 : BusSelector  OutputSignals=y_meas.h_geodetic,mode_sw.use_held_aero_obac_sw,y_meas.w_est,y_meas.NEh_dot,mode_sw.att_type,u_est,engines
  Gain1 : Gain  Orientation=left  Gain=use_variable_mass  ParameterDataType=sfix(16)  ParameterScaling=2^0  OutDataType=sfix(16)  OutScaling=2^0
  hold altitude : model_lib/hold input  SystemSampleTime=-1
  mass : DiscreteIntegrator  gainval=1  InitialCondition=MACH_mass_IC  SampleTime=-1  OutDataType=sfix(16)  OutScaling=2^0  ICPrevOutput=DiscIntNeverNeededParam  ICPrevScaledInput=DiscIntNeverNeededParam
  set scoped bus : model_lib/set scoped bus  SystemSampleTime=-1  vehicle_params=obac_params
  set scoped signals : model_lib/set scoped signals  SystemSampleTime=-1
  scoped_bus : Outport  OutDataType=sfix(16)  OutScaling=2^0
  wires:
  signal_bus/1 -> Bus Selector3/1
  Gain1/1 -> mass/1
  Bus Selector3/1 -> hold altitude/1  "<h_geodetic>"
  set scoped bus/2 -> Gain1/1
  set scoped bus/1 -> set scoped signals/1, scoped_bus/1
  mass/1 -> set scoped bus/7
  Bus Selector3/2 -> hold altitude/2  "<use_held_aero_obac_sw>"
  hold altitude/1 -> set scoped bus/1
  Bus Selector3/3 -> set scoped bus/2  "<w_est>"
  Bus Selector3/4 -> set scoped bus/3  "<NEh_dot>"
  Bus Selector3/5 -> set scoped bus/4  "<att_type>"
  Bus Selector3/6 -> set scoped bus/5  "<u_est>"
  Bus Selector3/7 -> set scoped bus/6  "<engines>"

== system main_sim_adapt/claw_main/state est ==
  u_old : Inport  OutDataType=sfix(16)  OutScaling=2^0
  sensors : Inport  Port=2  OutDataType=sfix(16)  OutScaling=2^0
  signal_bus : Inport  Port=3  OutDataType=sfix(16)  OutScaling=2^0
  Bus Creator : BusCreator  Inputs=12
  Bus Creator1 : BusCreator  Inputs=6
  Bus Selector : BusSelector  OutputSignals=mode_sw.reset_pos_sw,mode_sw.nav_enable_sw,mode_sw.wind_est_sw
  Bus Selector1 : BusSelector  OutputSignals=nav_ok,pqr,NED_dot,latlonh,e
  Bus Selector2 : BusSelector  OutputSignals=aero_env.Mach,aero_env.vel,aero_env.alpha,aero_env.beta,aero_env.uvw_rw,aero_env.qbar
  Bus Selector3 : BusSelector  OutputSignals=u_meas,seeker,accels_cg
  Logical Operator : Logic  AllPortsSameDT=off  OutDataTypeMode=boolean  OutDataTypeStr=boolean
  beta_360 : Fcn  Expr=atan2(u(2),u(1))
  cl model : models/gtm-obac  SystemSampleTime=-1
  process inputs : Subsystem
  process sensors : Subsystem
  wind estimator : Subsystem
  y_meas : Outport  OutDataType=sfix(16)  OutScaling=2^0
  x_est : Outport  Port=2  OutDataType=sfix(16)  OutScaling=2^0
  xdot_est : Outport  Port=3  OutDataType=sfix(16)  OutScaling=2^0
  u_est : Outport  Port=4  OutDataType=sfix(16)  OutScaling=2^0
  aero_env_est : Outport  Port=5  OutDataType=sfix(16)  OutScaling=2^0
  w_est_debug : Outport  Port=6  OutDataType=sfix(16)  OutScaling=2^0
  wires:
  sensors/1 -> Bus Selector3/1, process inputs/2(sensors), wind estimator/3(sensors), Bus Selector1/1
  wind estimator/1(w_est) -> cl model/3, Bus Creator/12  "w_est"
  process sensors/8(dircos) -> wind estimator/1(dircos), Bus Creator/11  "dircos"
  cl model/1 -> xdot_est/1
  process sensors/9(x_est) -> cl model/1, wind estimator/2(x), x_est/1
  signal_bus/1 -> Bus Selector/1
  Bus Selector/1 -> process sensors/1(reset_pos)  "<reset_pos_sw>"
  Bus Selector/3 -> wind estimator/5(wind_est_sw)  "<wind_est_sw>"
  process inputs/1(u_est) -> u_est/1, cl model/2, wind estimator/4(u)
  Bus Selector1/2 -> process sensors/3(pqr)  "<pqr>"
  Bus Selector1/3 -> process sensors/4(NED_dot)  "<NED_dot>"
  Bus Selector1/4 -> process sensors/5(latlonh)  "<latlonh>"
  Bus Selector1/5 -> process sensors/6(e)  "<e>"
  process sensors/2(h_geodetic) -> Bus Creator/5  "h_geodetic"
  process sensors/3(NEh_nav) -> Bus Creator/6  "NEh_nav"
  process sensors/4(nav_valid) -> Bus Creator/7  "nav_valid"
  process sensors/5(NEh_dot) -> Bus Creator/8  "NEh_dot"
  process sensors/1(vehicle_origin) -> Bus Creator/4  "vehicle_origin"
  process sensors/7(cvc_origin) -> Bus Creator/10  "cvc_origin"
  u_old/1 -> process inputs/1(u_old)
  wind estimator/2(w_est_debug) -> w_est_debug/1
  cl model/2 -> Bus Selector2/1
  Bus Creator1/1 -> aero_env_est/1
  Logical Operator/1 -> process sensors/2(nav_ok)
  Bus Selector1/1 -> Logical Operator/2  "<nav_ok>"
  Bus Selector/2 -> Logical Operator/1  "<nav_enable_sw>"
  Bus Selector2/5 -> beta_360/1  "<uvw_rw>"
  process sensors/6(dc_fltpath) -> Bus Creator/9  "dc_fltpath"
  beta_360/1 -> Bus Creator1/5  "beta_360"
  Bus Selector2/1 -> Bus Creator1/1  "<Mach>"
  Bus Selector2/2 -> Bus Creator1/2  "<vel>"
  Bus Selector2/3 -> Bus Creator1/3  "<alpha>"
  Bus Selector2/4 -> Bus Creator1/4  "<beta>"
  Bus Selector2/6 -> Bus Creator1/6  "<qbar>"
  Bus Selector3/1 -> Bus Creator/1  "<u_meas>"
  Bus Selector3/2 -> Bus Creator/2  "<seeker>"
  Bus Selector3/3 -> Bus Creator/3  "<accels_cg>"
  Bus Creator/1 -> y_meas/1

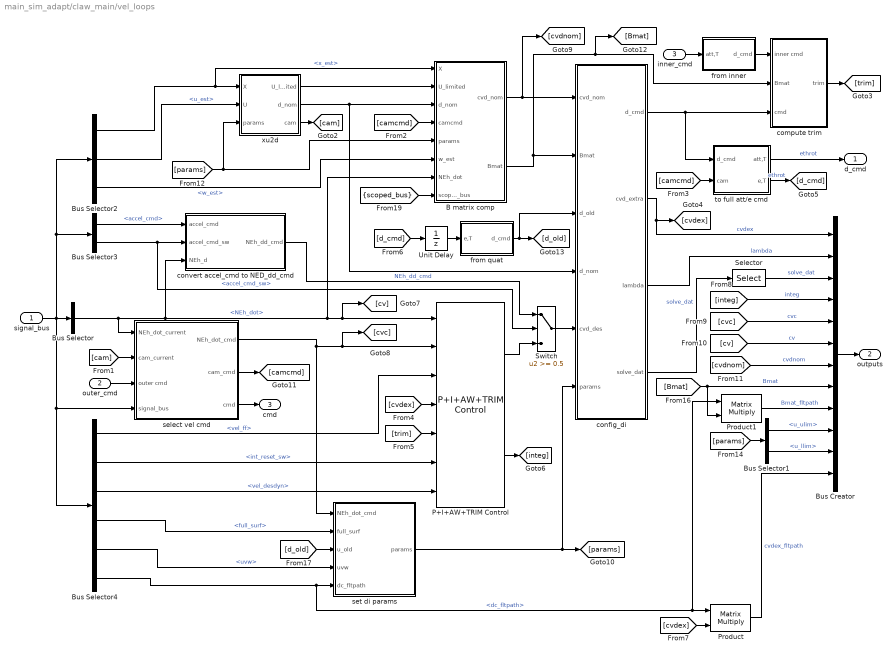
== system main_sim_adapt/claw_main/vel_loops ==
  signal_bus : Inport  OutDataType=sfix(16)  OutScaling=2^0
  outer_cmd : Inport  Port=2  OutDataType=sfix(16)  OutScaling=2^0
  inner_cmd : Inport  Port=3  OutDataType=sfix(16)  OutScaling=2^0
  B matrix comp : Subsystem
  Bus Creator : BusCreator  Inputs=12
  Bus Selector : BusSelector  OutputSignals=y_meas.NEh_dot
  Bus Selector1 : BusSelector  OutputSignals=u_ulim,u_llim
  Bus Selector2 : BusSelector  OutputSignals=x_est,u_est,y_meas.w_est
  Bus Selector3 : BusSelector  OutputSignals=control_params.accel_cmd,control_params.accel_cmd_sw
  Bus Selector4 : BusSelector  OutputSignals=feed_forward.vel_ff,mode_sw.int_reset_sw,control_params.vel_desdyn,full_surf,x_est.uvw,y_meas.dc_fltpath
  P+I+AW+TRIM Control : mach_lib/P+I+AW+TRIM Control  SystemSampleTime=-1
  Product : Product  Multiplication=Matrix(*)  OutDataType=sfix(16)  OutScaling=2^0  RndMeth=Zero
  Product1 : Product  Multiplication=Matrix(*)  OutDataType=sfix(16)  OutScaling=2^0  RndMeth=Zero
  Selector : Selector  NumberOfDimensions=2  InputPortWidth=MACH.num_u  IndexOptions=Index vector (dialog),Index vector (dialog)  Indices=1:9,1:2  OutputSizes=1
  Switch : Switch  Threshold=0.5
  Unit Delay : UnitDelay  X0=MACH_vel_uold_IC  SampleTime=-1
  compute trim : Subsystem
  config_di : Subsystem  BlockChoice=di_smn  mask{num_cv=MACH.vel_num_cv, num_u=MACH.vel_num_u, wght_cv_type=MACH.vel_wght_cv_type}
      link override di_smn/config_smn/smn_sfunc: sfunc_name=MACH.smn_sfunc_name
      link override di_smn/config_smn/smn_sfunc/S-Function: FunctionName=smn_sfunc_gam_mpass_epsposdef
      settings: AttributesFormatString=%<BlockChoice>  TemplateBlock=mach_lib/config_di  MemberBlocks=di_pseudoinv,di_smn
  convert accel_cmd to NED_dd_cmd : Subsystem  TreatAsAtomicUnit=on
  from inner : Subsystem
  from quat : Subsystem
  select vel cmd : Subsystem
  set di params : Subsystem
  to full att/e cmd : Subsystem
  xu2d : Subsystem
  d_cmd : Outport  OutDataType=sfix(16)  OutScaling=2^0
  outputs : Outport  Port=2  OutDataType=sfix(16)  OutScaling=2^0
  cmd : Outport  Port=3  OutDataType=sfix(16)  OutScaling=2^0
  wires:
  B matrix comp/2(Bmat) -> config_di/2(Bmat), compute trim/2(Bmat), [Bmat]
  to full att/e cmd/1(att,T) -> d_cmd/1  "ethrot"
  config_di/1(d_cmd) -> compute trim/3(cmd), to full att/e cmd/1(d_cmd)
  P+I+AW+TRIM Control/2 -> [integ]
  xu2d/2(d_nom) -> config_di/4(d_nom), B matrix comp/3(d_nom)
  Bus Selector/1 -> convert accel_cmd to NED_dd_cmd/3(NEh_d), B matrix comp/7(NEh_dot), P+I+AW+TRIM Control/1, [cv], select vel cmd/1(NEh_dot_current)  "<NEh_dot>"
  xu2d/3(cam) -> [cam]
  [cam] -> select vel cmd/2(cam_current)
  compute trim/1(trim) -> [trim]
  inner_cmd/1 -> from inner/1(att,T)
  from inner/1(d_cmd) -> compute trim/1(inner cmd)
  [camcmd] -> to full att/e cmd/2(cam)
  Bus Selector2/3 -> B matrix comp/6(w_est)  "<w_est>"
  [d_cmd] -> Unit Delay/1
  Unit Delay/1 -> from quat/1(e,T)
  set di params/1(params) -> [params], config_di/6(params)
  [params] -> xu2d/3(params), B matrix comp/5(params)
  xu2d/1(U_limited) -> B matrix comp/2(U_limited)
  [integ] -> Bus Creator/4  "integ"
  [cvc] -> Bus Creator/5  "cvc"
  [cv] -> Bus Creator/6  "cv"
  [cvdnom] -> Bus Creator/7  "cvdnom"
  [trim] -> P+I+AW+TRIM Control/5
  [cvdex] -> P+I+AW+TRIM Control/4
  Bus Selector4/2 -> P+I+AW+TRIM Control/6  "<int_reset_sw>"
  Bus Selector4/1 -> P+I+AW+TRIM Control/3  "<vel_ff>"
  B matrix comp/1(cvd_nom) -> [cvdnom], config_di/1(cvd_nom)
  [Bmat] -> Product1/2, Bus Creator/8  "Bmat"
  config_di/2(cvd_extra) -> [cvdex], Bus Creator/1  "cvdex"
  from quat/1(d_cmd) -> [d_old], config_di/3(d_old)
  Bus Selector4/4 -> set di params/2(full_surf)  "<full_surf>"
  Product/1 -> Bus Creator/12  "cvdex_fltpath"
  [params] -> Bus Selector1/1
  Bus Selector1/1 -> Bus Creator/10  "<u_ulim>"
  Bus Selector1/2 -> Bus Creator/11  "<u_llim>"
  [d_old] -> set di params/3(u_old)
  Bus Selector4/5 -> set di params/4(uvw)  "<uvw>"
  config_di/3(lambda) -> Bus Creator/2  "lambda"
  config_di/4(solve_dat) -> Selector/1  "solve_dat"
  [cvdex] -> Product/2
  Selector/1 -> Bus Creator/3  "solve_dat"
  [camcmd] -> B matrix comp/4(camcmd)
  [scoped_bus] -> B matrix comp/8(scoped_bus)
  Bus Selector2/1 -> xu2d/1(X), B matrix comp/1(X)  "<x_est>"
  Bus Selector2/2 -> xu2d/2(U)  "<u_est>"
  Bus Selector4/3 -> P+I+AW+TRIM Control/7  "<vel_desdyn>"
  Bus Selector3/1 -> convert accel_cmd to NED_dd_cmd/1(accel_cmd)  "<accel_cmd>"
  Switch/1 -> config_di/5(cvd_des)
  P+I+AW+TRIM Control/1 -> Switch/3
  convert accel_cmd to NED_dd_cmd/1(NEh_dd_cmd) -> Switch/1  "NEh_dd_cmd"
  signal_bus/1 -> Bus Selector/1, Bus Selector3/1, Bus Selector2/1, Bus Selector4/1, select vel cmd/4(signal_bus)
  Bus Selector3/2 -> convert accel_cmd to NED_dd_cmd/2(accel_cmd_sw), Switch/2  "<accel_cmd_sw>"
  Product1/1 -> Bus Creator/9  "Bmat_fltpath"
  Bus Selector4/6 -> Product/1, Product1/1, set di params/5(dc_fltpath)  "<dc_fltpath>"
  to full att/e cmd/2(e,T) -> [d_cmd]  "ethrot"
  outer_cmd/1 -> select vel cmd/3(outer cmd)
  select vel cmd/3(cmd) -> cmd/1
  select vel cmd/2(cam_cmd) -> [camcmd]
  select vel cmd/1(NEh_dot_cmd) -> set di params/1(NEh_dot_cmd), P+I+AW+TRIM Control/2, [cvc]
  Bus Creator/1 -> outputs/1

== system main_sim_adapt/vehicle_model/a/c model ==
  u : Inport  OutDataType=sfix(16)  OutScaling=2^0
  integrate_state : Inport  Port=2  OutDataType=sfix(16)  OutScaling=2^0
  NED_wind : Inport  Port=3  OutDataType=sfix(16)  OutScaling=2^0
  Logical Operator : Logic  Operator=NOT  AllPortsSameDT=off  OutDataTypeMode=boolean  OutDataTypeStr=boolean
  Product : Product  OutDataType=sfix(16)  OutScaling=2^0  RndMeth=Zero
  e mag error feedback : model_lib/e mag error feedback  SystemSampleTime=-1
  vehicle model : models/gtm-trac  SystemSampleTime=-1  vehicle_params=trac_params
  vehicle state integrator : Integrator  ExternalReset=level  InitialCondition=x_trac_IC
  x : Outport  OutDataType=sfix(16)  OutScaling=2^0
  xdot : Outport  Port=2  OutDataType=sfix(16)  OutScaling=2^0
  y : Outport  Port=3  OutDataType=sfix(16)  OutScaling=2^0
  wires:
  u/1 -> vehicle model/2
  vehicle state integrator/1 -> x/1, vehicle model/1, e mag error feedback/1
  integrate_state/1 -> Logical Operator/1, Product/2
  Product/1 -> xdot/1, vehicle state integrator/1
  Logical Operator/1 -> vehicle state integrator/2
  NED_wind/1 -> vehicle model/3
  vehicle model/2 -> y/1
  e mag error feedback/1 -> Product/1
  vehicle model/1 -> e mag error feedback/2

== system main_sim_adapt/vehicle_model/apply additional limits ==
  effector_limits_in : Inport  OutDataType=sfix(16)  OutScaling=2^0
  Bus Assignment : BusAssignment  AssignedSignals=u_ulim,u_llim
  Bus Selector : BusSelector  OutputSignals=u_ulim,u_llim
  throt out of fuel limits : model_lib/throt out of fuel limits  SystemSampleTime=-1
  effector_limits : Outport  OutDataType=sfix(16)  OutScaling=2^0
  wires:
  effector_limits_in/1 -> Bus Assignment/1, Bus Selector/1
  Bus Selector/1 -> throt out of fuel limits/1  "<u_ulim>"
  Bus Selector/2 -> throt out of fuel limits/2  "<u_llim>"
  Bus Assignment/1 -> effector_limits/1
  throt out of fuel limits/1 -> Bus Assignment/2
  throt out of fuel limits/2 -> Bus Assignment/3

== system main_sim_adapt/vehicle_model/set scoped signals ==
  note: Note: att_type is not actually
      | used by the trac
  output_bus : Inport  OutDataType=sfix(16)  OutScaling=2^0
  Bus Selector1 : BusSelector  OutputSignals=x,use_held_aero_trac_sw,NED_wind,xdot,u_servo,engines
  Constant2 : Constant  Value=MACH.att_type  OutDataType=sfix(16)  OutScaling=2^0
  Gain1 : Gain  Orientation=left  Gain=use_variable_mass  ParameterDataType=sfix(16)  ParameterScaling=2^0  OutDataType=sfix(16)  OutScaling=2^0
  NEh_dot : Selector  InputPortWidth=trac_params.num_x  IndexOptions=Index vector (dialog)  Indices=MACH.NEh_idx  OutputSizes=1
  h : Selector  InputPortWidth=MACH.num_x  IndexOptions=Index vector (dialog)  Indices=MACH.NEh_idx(3)  OutputSizes=1
  hold altitude : model_lib/hold input  SystemSampleTime=-1
  mass integrator : Integrator  InitialCondition=trac_params.mass_IC
  set scoped bus : model_lib/set scoped bus  SystemSampleTime=-1  vehicle_params=trac_params
  set scoped signals : model_lib/set scoped signals  SystemSampleTime=-1
  scoped_bus : Outport  OutDataType=sfix(16)  OutScaling=2^0
  wires:
  Bus Selector1/1 -> h/1  "<x>"
  NEh_dot/1 -> set scoped bus/3
  Bus Selector1/3 -> set scoped bus/2  "<NED_wind>"
  Bus Selector1/5 -> set scoped bus/5  "<u_servo>"
  mass integrator/1 -> set scoped bus/7
  set scoped bus/2 -> Gain1/1
  Gain1/1 -> mass integrator/1
  hold altitude/1 -> set scoped bus/1
  h/1 -> hold altitude/1
  Bus Selector1/2 -> hold altitude/2  "<use_held_aero_trac_sw>"
  set scoped bus/1 -> set scoped signals/1, scoped_bus/1
  Constant2/1 -> set scoped bus/4
  Bus Selector1/4 -> NEh_dot/1  "<xdot>"
  output_bus/1 -> Bus Selector1/1
  Bus Selector1/6 -> set scoped bus/6  "<engines>"

== system main_sim_adapt/vehicle_model/target/seeker model ==
  output_bus : Inport  OutDataType=sfix(16)  OutScaling=2^0
  Bus Selector : BusSelector  OutputSignals=x,xdot
  Bus Selector1 : BusSelector  OutputSignals=LOS_rate,aux_info.azimuth,aux_info.elevation,aux_info.Rground,aux_info.Rslant
  Constant2 : Constant  Value=target_vel_IC  OutDataType=sfix(16)  OutScaling=2^0
  NEh : Selector  InputPortWidth=MACH.num_x  IndexOptions=Index vector (dialog)  Indices=MACH.NEh_idx  OutputSizes=1
  NEh_dot : Selector  InputPortWidth=MACH.num_x  IndexOptions=Index vector (dialog)  Indices=MACH.NEh_idx  OutputSizes=1
  seeker model : Subsystem
  seeker scope : Scope  NumInputPorts=5
      settings: YMin=-1.75~-3.5~-1.75~0~0  YMax=0.25~0.5~0~450000~550000
  target position integrator : Integrator  InitialCondition=target_pos_IC
  seeker : Outport  OutDataType=sfix(16)  OutScaling=2^0
  wires:
  Constant2/1 -> target position integrator/1, seeker model/2(NEh_d_target)
  target position integrator/1 -> seeker model/1(NEh_target)
  NEh/1 -> seeker model/3(NEh)
  NEh_dot/1 -> seeker model/4(NEh_d)
  seeker model/1(seeker) -> seeker/1, Bus Selector1/1
  output_bus/1 -> Bus Selector/1
  Bus Selector/1 -> NEh/1  "<x>"
  Bus Selector/2 -> NEh_dot/1  "<xdot>"
  Bus Selector1/2 -> seeker scope/2  "<azimuth>"
  Bus Selector1/3 -> seeker scope/3  "<elevation>"
  Bus Selector1/4 -> seeker scope/4  "<Rground>"
  Bus Selector1/5 -> seeker scope/5  "<Rslant>"
  Bus Selector1/1 -> seeker scope/1  "<LOS_rate>"

== system main_sim_adapt/claw_main/att_loops/P+I+AW+TRIM Control ==
  cv : Inport  OutDataType=sfix(16)  OutScaling=2^0
  cv cmd : Inport  Port=2  OutDataType=sfix(16)  OutScaling=2^0
  cvd ff : Inport  Port=3  OutDataType=sfix(16)  OutScaling=2^0
  cvdot extra : Inport  Port=4  OutDataType=sfix(16)  OutScaling=2^0
  trim : Inport  Port=5  OutDataType=sfix(16)  OutScaling=2^0
  reset : Inport  Port=6  OutDataType=sfix(16)  OutScaling=2^0
  x0 : Inport  Port=7  OutDataType=sfix(16)  OutScaling=2^0
  Dot Product2 : simulink/Math Operations/Dot Product  InputSameDT=on  OutDataType=sfix(16)  OutScaling=2^-10  DoSatur=off
  P+I+AW+TRIM Control : mach_lib/P+I+AW+TRIM Control  SystemSampleTime=-1
  Product2 : Product  OutDataType=sfix(16)  OutScaling=2^0  SaturateOnIntegerOverflow=on  InputSameDT=on  OutDataTypeStr=Inherit: Same as first input
  Sum : Sum  Inputs=-+|  OutDataType=sfix(16)  OutScaling=2^0  SaturateOnIntegerOverflow=on
  Unit Delay1 : UnitDelay  SampleTime=-1
  fe : Gain  Gain=MACH.att_fe  ParameterDataType=sfix(16)  ParameterScaling=2^0  OutDataType=sfix(16)  OutScaling=2^0  SaturateOnIntegerOverflow=on  OutDataTypeStr=Inherit: Same as input  ParamDataTypeStr=Inherit: Same as input
  cvdot des : Outport  OutDataType=sfix(16)  OutScaling=2^0
  int state : Outport  Port=2  OutDataType=sfix(16)  OutScaling=2^0
  wires:
  cvd ff/1 -> P+I+AW+TRIM Control/3
  cvdot extra/1 -> P+I+AW+TRIM Control/4
  Sum/1 -> P+I+AW+TRIM Control/5
  reset/1 -> P+I+AW+TRIM Control/6
  x0/1 -> P+I+AW+TRIM Control/7
  fe/1 -> Sum/1
  trim/1 -> Sum/2
  Product2/1 -> fe/1
  Unit Delay1/1 -> Dot Product2/2
  Dot Product2/1 -> Product2/2
  P+I+AW+TRIM Control/2 -> int state/1
  P+I+AW+TRIM Control/1 -> Unit Delay1/1, cvdot des/1
  cv cmd/1 -> P+I+AW+TRIM Control/2
  cv/1 -> Product2/1, Dot Product2/1, P+I+AW+TRIM Control/1
